simulink model "MRA"  (R2026a)
settings: Solver=ode4  StopTime=5  FixedStep=0.002
values from neighbouring files (symbols this model uses):
  c = 5    [MRA_ode45.m]
  k = 400    [MRA_ode45.m]
  m = 1    [MRA_ode45.m]
settings Model: Creator=20808  LastModifiedBy=20808

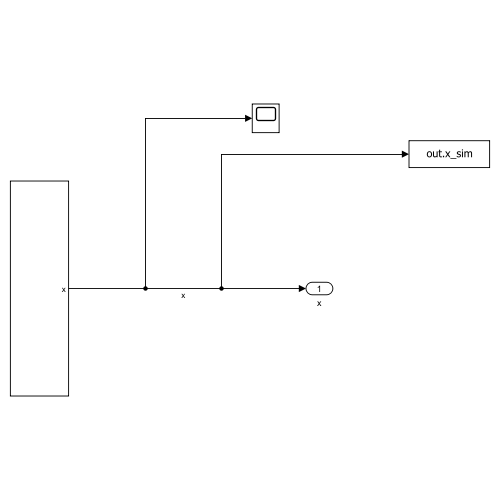
[thumbnail: Simulink's stored preview of the top-level diagram]
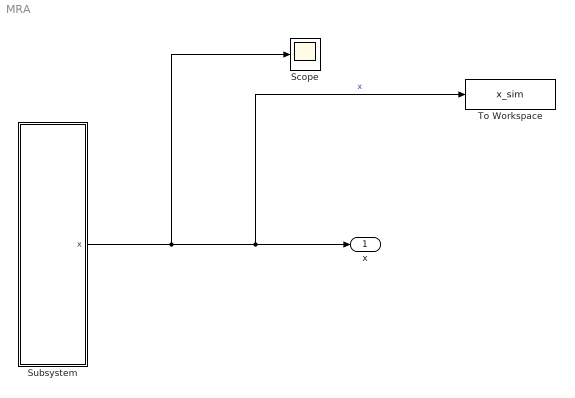
== system MRA ==
  Scope : Scope
  Subsystem : Subsystem
  To Workspace : ToWorkspace  VariableName=x_sim  SaveFormat=Timeseries  SampleTime=-1
  x : Outport
  wires:
  Subsystem/1(x) -> Scope/1, To Workspace/1, x/1  "x"

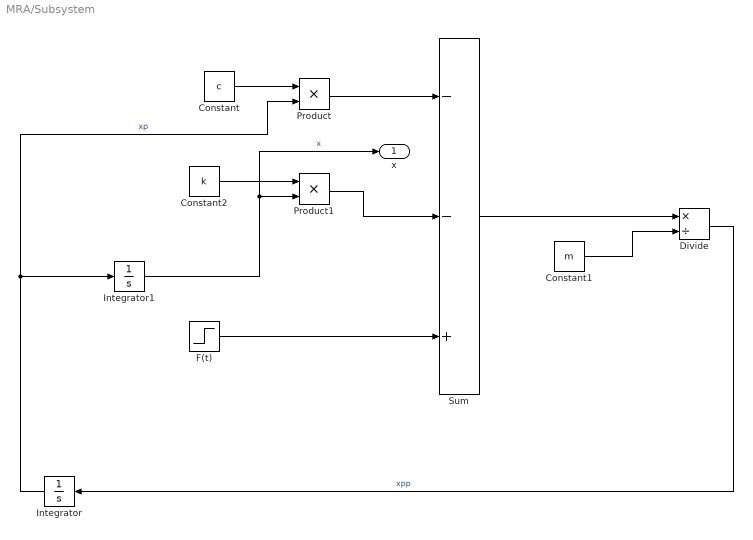
== system MRA/Subsystem ==
  Constant : Constant  Value=c
  Constant1 : Constant  Value=m
  Constant2 : Constant  Value=k
  Divide : Product  Inputs=*/
  F(t) : Step  Time=0.25  FinalValue=10  SampleTime=0
  Integrator : Integrator
  Integrator1 : Integrator
  Product : Product
  Product1 : Product
  Sum : Sum  Inputs=--+
  x : Outport
  wires:
  Product1/1 -> Sum/2
  Constant1/1 -> Divide/2
  Sum/1 -> Divide/1
  Divide/1 -> Integrator/1  "xpp"
  Integrator/1 -> Integrator1/1, Product/2  "xp"
  Product/1 -> Sum/1
  Integrator1/1 -> x/1, Product1/2  "x"
  Constant/1 -> Product/1
  Constant2/1 -> Product1/1
  F(t)/1 -> Sum/3
